simulink model "act3"  (R2020a)
settings: Solver=ode1  StartTime=0.0  StopTime=10.0  FixedStep=1e-2  RelTol=1e-3
values from neighbouring files (symbols this model uses):
  a_1 = 1    [act1_script.m]
  a_2 = 2    [act1_script.m]
undefined symbols (not defined in the file or in its folder): c
settings Model: Creator=Jorjolo  LastModifiedBy=Jorjolo

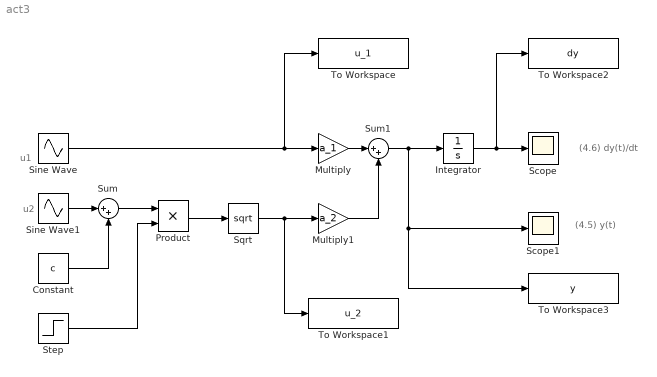
== system act3 ==
  note: (4.5)
      | y(t)
  note: (4.6)
      | dy(t)/dt
  note: u2
  note: u1
  Constant : Constant  Value=c
  Integrator : Integrator
  Multiply : Gain  Gain=a_1
  Multiply1 : Gain  Gain=a_2
  Product : Product
  Scope : Scope
  Scope1 : Scope
  Sine Wave : Sin  Frequency=100  SampleTime=0
  Sine Wave1 : Sin  Amplitude=1.5  Frequency=10  SampleTime=0
  Sqrt : Sqrt  SaturateOnIntegerOverflow=on
  Step : Step  Time=0  SampleTime=0
  Sum : Sum  Inputs=|++
  Sum1 : Sum  Inputs=|++
  To Workspace : ToWorkspace  VariableName=u_1  SampleTime=1e-2
  To Workspace1 : ToWorkspace  VariableName=u_2  SampleTime=1e-2
  To Workspace2 : ToWorkspace  VariableName=dy  SampleTime=1e-2
  To Workspace3 : ToWorkspace  VariableName=y  SampleTime=-1
  wires:
  Step/1 -> Product/2
  Product/1 -> Sqrt/1
  Sine Wave/1 -> Multiply/1, To Workspace/1
  Sine Wave1/1 -> Sum/1
  Constant/1 -> Sum/2
  Sum/1 -> Product/1
  Multiply/1 -> Sum1/1
  Multiply1/1 -> Sum1/2
  Sqrt/1 -> To Workspace1/1, Multiply1/1
  Sum1/1 -> To Workspace3/1, Scope1/1, Integrator/1
  Integrator/1 -> To Workspace2/1, Scope/1
